simulink model "APP_MyApplication"  (R2018b)
settings: Solver=VariableStepDiscrete  StartTime=0.0  StopTime=10  RelTol=1e-3
PreLoadFcn:
  | if(exist('MBDS_ModelCallback', 'file')), MBDS_ModelCallback('PreLoad'); end;
PostLoadFcn:
  | if(exist('MBDS_ModelCallback', 'file')), MBDS_ModelCallback('PostLoad'); end;
InitFcn:
  | if(exist('MBDS_ModelCallback', 'file')), MBDS_ModelCallback('Init'); end;
StartFcn:
  | if(exist('MBDS_ModelCallback', 'file')), MBDS_ModelCallback('Start'); end;
StopFcn:
  | if(exist('MBDS_ModelCallback', 'file')), MBDS_ModelCallback('Stop'); end;
undefined symbols (not defined in the file): sigbuilder_block, Ts
libraries: KIBES_Signal x499, simulink x8
(part 8 of 10)

== system APP_MyApplication/Model/APP_MyApplication_/EEProm/TimerPulse ==
  note: Timer Pulse
  bo_Enable : Inport  OutDataTypeStr=boolean
  EdgeRising : Subsystem  InitFcn=|  mask(EdgeRising){MBDS_LibraryBlock=on, R_Enabled=off, IV_Enabled=off, IV=0, MBDS_BlockVersion=05.32}
      | if(exist('MBDS_BlockCallback', 'file'))
      |    MBDS_BlockCallback('Update', gcb);
      | end
      mask prompts: MBDS_LibraryBlock "MBDS library block"; R_Enabled "Show R port"; IV_Enabled "Show IV port"; IV "Initial value (IV):"; MBDS_BlockVersion "Block version:"
      mask help: The output indicates true if the input value changes from false to true.
      mask init: same as APP_MyApplication/Model/APP_MyApplication_/OR
      mask Help: eval(['open([workdir(''library_dir:''),''\Blockset\help\'',get_param(gcb,''MaskType''),''.html''])'])
      mask Callback R_Enabled:
      | % Update mask parameter dialog
      | if(exist('MBDS_BlockCallback', 'file'))
      |    MBDS_BlockCallback('R_Enabled', gcb);
      | end
      mask Callback IV_Enabled:
      | % Update mask parameter dialog
      | if(exist('MBDS_BlockCallback', 'file'))
      |    MBDS_BlockCallback('IV_Enabled', gcb);
      | end
      mask Callback IV:
      | % Adopt Value
      | if(exist('MBDS_BlockCallback', 'file'))
      |    MBDS_BlockCallback('IV', gcb);
      | end
      mask DialogControl ParameterTabVar0 Prompt: Main
      mask DialogControl ParameterTabVar01 Prompt: Version
      mask Display:
      | % Show icon or block text
      | if(exist('EdgeRising.tif', 'file'))
      |    image('EdgeRising.tif', [0.295739348370927 0.17 0.378947368421053 0.66]);
      |    disp('')
      | else
      |    disp(sprintf('Rising\nEdge\nDetection'));
      | end
      | 
      | % Display port labels
      | port_label('input', 1, 'u');
      | port_label('output', 1, 'y');
  TimeSource : Subsystem  InitFcn=|  mask(TimeSource){MBDS_LibraryBlock=on, InputValue=10ms, MBDS_BlockVersion=07.21.04}
      | if(exist('MBDS_BlockCallback', 'file'))
      |    MBDS_BlockCallback('Update', gcb);
      | end
      mask prompts: MBDS_LibraryBlock "MBDS Library Block"; InputValue "Constant value:"; MBDS_BlockVersion "Block version:"
      mask help: This block outputs a constant time signal based on a uint32 data type. Specify the time by the 'Constant value' parameter. Comply to the format: 1d2h3m4s5ms, for example 12d10h34m4s231ms, 1s500ms or 2h1s.
      mask init: same as APP_MyApplication/Model/APP_MyApplication_/TimerPulse/TimeSource
      mask Help: eval(['open([workdir(''Library_Dir:''),''\Blockset\Help\'',get_param(gcb,''MaskType''),''.html''])'])
      mask DialogControl ParameterTabVar0 Prompt: Main
      mask DialogControl ParameterTabVar01 Prompt: Version
      mask Display: disp([' ',Text,' ']);
  Timer_RE1 : Subsystem  InitFcn=|  mask(Timer_RE){MBDS_LibraryBlock=on, dT_Enabled=off, dT=1000*Ts, E_Enabled=off, R_Enabled=on, IV_Enabled=on, IV=0, y_Enabled=on, x_Enabled=off, OutDataTypeStr=Inherit: Inherit via back propagation, MBDS_BlockVersion=05.20}
      | if(exist('MBDS_BlockCallback', 'file'))
      |    MBDS_BlockCallback('Update', gcb);
      | end
      mask prompts: MBDS_LibraryBlock "MBDS library block"; dT_Enabled "Show dT port"; dT "Sample rate (dT):"; E_Enabled "Show E port"; R_Enabled "Show R port"; IV_Enabled "Show IV port"; IV "Initial value (IV):"; y_Enabled "Show y port"; x_Enabled "Show x port"; OutDataTypeStr "Output data type:"; MBDS_BlockVersion "Block version:"
      mask help: The block indicates true, if the initial time IV has not passed since the last reset of the block. Reset can only be performed, if the counter has run down to zero.
      mask init: same as APP_MyApplication/Model/APP_MyApplication_/OR
      settings: AttributesFormatString=dT = %<dT>
      mask Help: eval(['open([workdir(''library_dir:''),''\Blockset\help\'',get_param(gcb,''MaskType''),''.html''])'])
      mask Callback dT_Enabled:
      | % Update mask parameter dialog
      | if(exist('MBDS_BlockCallback', 'file'))
      |    MBDS_BlockCallback('dT_Enabled', gcb);
      | end
      mask Callback dT:
      | % Adopt Value
      | if(exist('MBDS_BlockCallback', 'file'))
      |    MBDS_BlockCallback('dT', gcb);
      | end
      mask Callback R_Enabled:
      | % Update mask parameter dialog
      | if(exist('MBDS_BlockCallback', 'file'))
      |    MBDS_BlockCallback('R_Enabled', gcb);
      | end
      mask Callback IV_Enabled:
      | % Update mask parameter dialog
      | if(exist('MBDS_BlockCallback', 'file'))
      |    MBDS_BlockCallback('IV_Enabled', gcb);
      | end
      mask Callback IV:
      | % Adopt Value
      | if(exist('MBDS_BlockCallback', 'file'))
      |    MBDS_BlockCallback('IV', gcb);
      | end
      mask Callback y_Enabled:
      | % Update mask parameter dialog
      | if(exist('MBDS_BlockCallback', 'file'))
      |    MBDS_BlockCallback('y_Enabled', gcb);
      | end
      mask Callback x_Enabled:
      | % Update mask parameter dialog
      | if(exist('MBDS_BlockCallback', 'file'))
      |    MBDS_BlockCallback('x_Enabled', gcb);
      | end
      mask TypeOptions OutDataTypeStr: Inherit: Inherit via back propagation | int8 | uint8 | int16 | uint16 | int32 | uint32
      mask Callback OutDataTypeStr:
      | % Configure data type
      | if(exist('MBDS_BlockCallback', 'file'))
      |    MBDS_BlockCallback('OutDataTypeStr', gcb);
      | end
      mask DialogControl ParameterTabVar0 Prompt: Main
      mask DialogControl ParameterTabVar01 Prompt: Signal Attributes
      mask DialogControl ParameterTabVar012 Prompt: Version
      mask Display:
      | % Show icon or block text
      | if(exist('Timer.tif', 'file'))
      |    image('Timer.tif', [0.295739348370927 0.17 0.378947368421053 0.66]);
      |    disp('')
      | else
      |    disp(sprintf('Timer'));
      | end
      | 
      | % Display port labels
      | port_label('input', 1, 'R');
      | port_label('input', 2, 'IV');
      | port_label('output', 1, 'y');
  bo_Pulse : Outport
  wires:
  EdgeRising/1(y) -> Timer_RE1/1(R)
  Timer_RE1/1(y) -> bo_Pulse/1
  bo_Enable/1 -> EdgeRising/1(u)
  TimeSource/1(Out) -> Timer_RE1/2(IV)

== system APP_MyApplication/Model/APP_MyApplication_/EEProm/TimerPulse1 ==
  note: Timer Pulse
  bo_Enable : Inport  OutDataTypeStr=boolean
  EdgeRising : Subsystem  InitFcn=|  mask(EdgeRising){MBDS_LibraryBlock=on, R_Enabled=off, IV_Enabled=off, IV=0, MBDS_BlockVersion=05.32}
      | if(exist('MBDS_BlockCallback', 'file'))
      |    MBDS_BlockCallback('Update', gcb);
      | end
      mask prompts: MBDS_LibraryBlock "MBDS library block"; R_Enabled "Show R port"; IV_Enabled "Show IV port"; IV "Initial value (IV):"; MBDS_BlockVersion "Block version:"
      mask help: The output indicates true if the input value changes from false to true.
      mask init: same as APP_MyApplication/Model/APP_MyApplication_/OR
      mask Help: eval(['open([workdir(''library_dir:''),''\Blockset\help\'',get_param(gcb,''MaskType''),''.html''])'])
      mask Callback R_Enabled:
      | % Update mask parameter dialog
      | if(exist('MBDS_BlockCallback', 'file'))
      |    MBDS_BlockCallback('R_Enabled', gcb);
      | end
      mask Callback IV_Enabled:
      | % Update mask parameter dialog
      | if(exist('MBDS_BlockCallback', 'file'))
      |    MBDS_BlockCallback('IV_Enabled', gcb);
      | end
      mask Callback IV:
      | % Adopt Value
      | if(exist('MBDS_BlockCallback', 'file'))
      |    MBDS_BlockCallback('IV', gcb);
      | end
      mask DialogControl ParameterTabVar0 Prompt: Main
      mask DialogControl ParameterTabVar01 Prompt: Version
      mask Display:
      | % Show icon or block text
      | if(exist('EdgeRising.tif', 'file'))
      |    image('EdgeRising.tif', [0.295739348370927 0.17 0.378947368421053 0.66]);
      |    disp('')
      | else
      |    disp(sprintf('Rising\nEdge\nDetection'));
      | end
      | 
      | % Display port labels
      | port_label('input', 1, 'u');
      | port_label('output', 1, 'y');
  TimeSource : Subsystem  InitFcn=|  mask(TimeSource){MBDS_LibraryBlock=on, InputValue=10ms, MBDS_BlockVersion=07.21.04}
      | if(exist('MBDS_BlockCallback', 'file'))
      |    MBDS_BlockCallback('Update', gcb);
      | end
      mask prompts: MBDS_LibraryBlock "MBDS Library Block"; InputValue "Constant value:"; MBDS_BlockVersion "Block version:"
      mask help: This block outputs a constant time signal based on a uint32 data type. Specify the time by the 'Constant value' parameter. Comply to the format: 1d2h3m4s5ms, for example 12d10h34m4s231ms, 1s500ms or 2h1s.
      mask init: same as APP_MyApplication/Model/APP_MyApplication_/TimerPulse/TimeSource
      mask Help: eval(['open([workdir(''Library_Dir:''),''\Blockset\Help\'',get_param(gcb,''MaskType''),''.html''])'])
      mask DialogControl ParameterTabVar0 Prompt: Main
      mask DialogControl ParameterTabVar01 Prompt: Version
      mask Display: disp([' ',Text,' ']);
  Timer_RE1 : Subsystem  InitFcn=|  mask(Timer_RE){MBDS_LibraryBlock=on, dT_Enabled=off, dT=1000*Ts, E_Enabled=off, R_Enabled=on, IV_Enabled=on, IV=0, y_Enabled=on, x_Enabled=off, OutDataTypeStr=Inherit: Inherit via back propagation, MBDS_BlockVersion=05.20}
      | if(exist('MBDS_BlockCallback', 'file'))
      |    MBDS_BlockCallback('Update', gcb);
      | end
      mask prompts: MBDS_LibraryBlock "MBDS library block"; dT_Enabled "Show dT port"; dT "Sample rate (dT):"; E_Enabled "Show E port"; R_Enabled "Show R port"; IV_Enabled "Show IV port"; IV "Initial value (IV):"; y_Enabled "Show y port"; x_Enabled "Show x port"; OutDataTypeStr "Output data type:"; MBDS_BlockVersion "Block version:"
      mask help: The block indicates true, if the initial time IV has not passed since the last reset of the block. Reset can only be performed, if the counter has run down to zero.
      mask init: same as APP_MyApplication/Model/APP_MyApplication_/OR
      settings: AttributesFormatString=dT = %<dT>
      mask Help: eval(['open([workdir(''library_dir:''),''\Blockset\help\'',get_param(gcb,''MaskType''),''.html''])'])
      mask Callback dT_Enabled:
      | % Update mask parameter dialog
      | if(exist('MBDS_BlockCallback', 'file'))
      |    MBDS_BlockCallback('dT_Enabled', gcb);
      | end
      mask Callback dT:
      | % Adopt Value
      | if(exist('MBDS_BlockCallback', 'file'))
      |    MBDS_BlockCallback('dT', gcb);
      | end
      mask Callback R_Enabled:
      | % Update mask parameter dialog
      | if(exist('MBDS_BlockCallback', 'file'))
      |    MBDS_BlockCallback('R_Enabled', gcb);
      | end
      mask Callback IV_Enabled:
      | % Update mask parameter dialog
      | if(exist('MBDS_BlockCallback', 'file'))
      |    MBDS_BlockCallback('IV_Enabled', gcb);
      | end
      mask Callback IV:
      | % Adopt Value
      | if(exist('MBDS_BlockCallback', 'file'))
      |    MBDS_BlockCallback('IV', gcb);
      | end
      mask Callback y_Enabled:
      | % Update mask parameter dialog
      | if(exist('MBDS_BlockCallback', 'file'))
      |    MBDS_BlockCallback('y_Enabled', gcb);
      | end
      mask Callback x_Enabled:
      | % Update mask parameter dialog
      | if(exist('MBDS_BlockCallback', 'file'))
      |    MBDS_BlockCallback('x_Enabled', gcb);
      | end
      mask TypeOptions OutDataTypeStr: Inherit: Inherit via back propagation | int8 | uint8 | int16 | uint16 | int32 | uint32
      mask Callback OutDataTypeStr:
      | % Configure data type
      | if(exist('MBDS_BlockCallback', 'file'))
      |    MBDS_BlockCallback('OutDataTypeStr', gcb);
      | end
      mask DialogControl ParameterTabVar0 Prompt: Main
      mask DialogControl ParameterTabVar01 Prompt: Signal Attributes
      mask DialogControl ParameterTabVar012 Prompt: Version
      mask Display:
      | % Show icon or block text
      | if(exist('Timer.tif', 'file'))
      |    image('Timer.tif', [0.295739348370927 0.17 0.378947368421053 0.66]);
      |    disp('')
      | else
      |    disp(sprintf('Timer'));
      | end
      | 
      | % Display port labels
      | port_label('input', 1, 'R');
      | port_label('input', 2, 'IV');
      | port_label('output', 1, 'y');
  bo_Pulse : Outport
  wires:
  EdgeRising/1(y) -> Timer_RE1/1(R)
  Timer_RE1/1(y) -> bo_Pulse/1
  bo_Enable/1 -> EdgeRising/1(u)
  TimeSource/1(Out) -> Timer_RE1/2(IV)

== system APP_MyApplication/Model/APP_MyApplication_/TimerPulse/EdgeRising ==
  note: EdgeRising
  u : Inport  OutDataTypeStr=boolean
  Data Type Duplicate : DataTypeDuplicate
  IV : Constant  Value=0  OutDataTypeStr=Inherit: Inherit via back propagation
  NoReset : Subsystem
  R : Constant  Value=0  OutDataTypeStr=boolean
  Relational Operator : RelationalOperator  Operator=<  OutDataTypeStr=boolean  RndMeth=Nearest  InputSameDT=on
  Unit Delay : UnitDelay  SampleTime=-1
  y : Outport
  wires:
  IV/1 -> NoReset/1(Unused1), Data Type Duplicate/2
  u/1 -> Unit Delay/1, Relational Operator/2, Data Type Duplicate/1
  R/1 -> NoReset/2(Unused2)
  NoReset/1(y) -> Relational Operator/1
  Unit Delay/1 -> NoReset/3(u)
  Relational Operator/1 -> y/1

== system APP_MyApplication/Model/APP_MyApplication_/TimerPulse/TimeSource ==
  note: TimeSource
  Constant : Constant  Value=Value  OutDataTypeStr=uint32  LockScale=on
  Out : Outport
  wires:
  Constant/1 -> Out/1

== system APP_MyApplication/Model/APP_MyApplication_/TimerPulse/Timer_RE1 ==
  note: Timer_RE
  R : Inport  OutDataTypeStr=boolean
  IV : Inport  Port=2
  Constant : Constant  Value=0  OutDataTypeStr=Inherit: Inherit via back propagation
  Constant1 : Constant  Value=0  OutDataTypeStr=Inherit: Inherit via back propagation
  Constant2 : Constant  Value=0  OutDataTypeStr=Inherit: Inherit via back propagation
  Data Type Duplicate : DataTypeDuplicate  NumInputPorts=3
  DoubleReset : Subsystem
  E : Constant  OutDataTypeStr=boolean
  NoEnable : Subsystem
  Relational Operator : RelationalOperator  Operator=<=  OutDataTypeStr=boolean  RndMeth=Nearest
  Relational Operator1 : RelationalOperator  Operator=>  OutDataTypeStr=boolean  RndMeth=Nearest
  Relational Operator2 : RelationalOperator  Operator=>  OutDataTypeStr=boolean  RndMeth=Nearest  InputSameDT=on
  Subtract : Sum  Inputs=+-  OutDataTypeStr=Inherit: Inherit via back propagation
  Switch1 : Switch  Criteria=u2 ~= 0  OutDataTypeStr=Inherit: Inherit via back propagation
  Unit Delay : UnitDelay  SampleTime=-1
  dT : Constant  Value=1000*Ts  OutDataTypeStr=Inherit: Inherit via back propagation
  x : Terminator
  y : Outport
  wires:
  R/1 -> DoubleReset/2(R1)
  E/1 -> NoEnable/2(Unused1)
  IV/1 -> Data Type Duplicate/1, DoubleReset/1(IV)
  Relational Operator/1 -> DoubleReset/3(R2)
  DoubleReset/1(y) -> Relational Operator2/1, Unit Delay/1, x/1, Data Type Duplicate/3
  Constant2/1 -> Relational Operator2/2
  Constant/1 -> Switch1/3
  Subtract/1 -> Switch1/1
  Relational Operator1/1 -> Switch1/2
  Switch1/1 -> NoEnable/1(u)
  dT/1 -> Subtract/2, Relational Operator1/2
  Unit Delay/1 -> NoEnable/3(Unused2), Relational Operator1/1, Subtract/1, Relational Operator/1, Data Type Duplicate/2
  Constant1/1 -> Relational Operator/2
  NoEnable/1(y) -> DoubleReset/4(u)
  Relational Operator2/1 -> y/1

== system APP_MyApplication/Model/APP_MyApplication_/UDS Service/RSFlipFlop ==
  note: RSFlipFlop
  SET : Inport  OutDataTypeStr=boolean
  RST : Inport  Port=2  OutDataTypeStr=boolean
  Constant : Constant  Value=0  OutDataTypeStr=Inherit: Inherit via back propagation
  Constant1 : Constant  OutDataTypeStr=Inherit: Inherit via back propagation
  Data Type Duplicate : DataTypeDuplicate  NumInputPorts=3
  Logical Operator : Logic  Operator=NOT  AllPortsSameDT=off  OutDataTypeStr=boolean
  Switch1 : Switch  Criteria=u2 ~= 0  OutDataTypeStr=Inherit: Inherit via back propagation
  Switch2 : Switch  Criteria=u2 ~= 0  OutDataTypeStr=Inherit: Inherit via back propagation
  Unit Delay : UnitDelay  SampleTime=-1
  Q : Outport
  ~Q : Outport  Port=2
  wires:
  Switch1/1 -> Q/1, Data Type Duplicate/3, Unit Delay/1, Logical Operator/1
  Constant/1 -> Switch1/1
  RST/1 -> Data Type Duplicate/2, Switch1/2
  SET/1 -> Data Type Duplicate/1, Switch2/2
  Constant1/1 -> Switch2/1
  Switch2/1 -> Switch1/3
  Logical Operator/1 -> ~Q/1
  Unit Delay/1 -> Switch2/3

== system APP_MyApplication/Model/APP_MyApplication_/DTC/DateTimeDisassemble/CheckIfTimeDataIsValid ==
  note: 2099-12-31-23:59:59
  note: Check if time data is valid
  u32_DateTime : Inport  OutDataTypeStr=uint32
  Constant14 : Constant  Value=4102444799  OutDataTypeStr=uint32
  Relational Operator : RelationalOperator  Operator=<=  OutDataTypeStr=boolean  RndMeth=Nearest
  bo_ENO : Outport  OutDataTypeStr=boolean
  wires:
  Constant14/1 -> Relational Operator/2
  u32_DateTime/1 -> Relational Operator/1
  Relational Operator/1 -> bo_ENO/1

== system APP_MyApplication/Model/APP_MyApplication_/DTC/DateTimeDisassemble/CheckLeapYearsAndRemainingDays ==
  note: Year
  note: Check leap year and calculate remaining days in current year
  note: avoid overflow
  u16_NrOfDays : Inport  OutDataTypeStr=uint16
  Add3 : Sum  Inputs=++-  OutDataTypeStr=uint16
  CalculateLeapYearsSince1970 : Subsystem
  CalculateRemainingDays : Subsystem
  CheckIfCorrectedTempYearIsLeap : Subsystem
  CheckIfTempYearIsCorrect : Subsystem
  CheckLeapYear : Subsystem
  Constant2 : Constant  OutDataTypeStr=uint16
  Constant6 : Constant  Value=0  OutDataTypeStr=uint16
  DaysPerNonLeapYear : Constant  Value=365  OutDataTypeStr=uint16
  Math Function3 : Math  Operator=rem  OutputSignalType=real  SaturateOnIntegerOverflow=on
  Relational Operator1 : RelationalOperator  Operator===  OutDataTypeStr=boolean  RndMeth=Nearest  InputSameDT=on
  Switch1 : Switch  Criteria=u2 ~= 0  OutDataTypeStr=uint16
  u16_TempDate : Outport  OutDataTypeStr=uint16
  u16_Year : Outport  Port=2  OutDataTypeStr=uint16
  bo_LeapYear : Outport  Port=3  OutDataTypeStr=boolean
  wires:
  u16_NrOfDays/1 -> CalculateLeapYearsSince1970/1(u16_NrOfDays), Math Function3/1
  DaysPerNonLeapYear/1 -> CalculateRemainingDays/5(u16_DaysPerCommonYear), Math Function3/2, CalculateLeapYearsSince1970/2(u16_DaysPerCommonYear)
  Math Function3/1 -> CalculateRemainingDays/3(u16_TempRemainingDays), CheckIfTempYearIsCorrect/1(u16_TempRemainingDays)
  Switch1/1 -> CheckLeapYear/1(u16_Year), u16_Year/1
  CalculateLeapYearsSince1970/2(u16_TempYear) -> Switch1/1, Add3/2, Relational Operator1/2
  Add3/1 -> Switch1/3, CheckIfCorrectedTempYearIsLeap/1(u16_CorrectedTempYear)
  CheckLeapYear/1(bo_LeapYear) -> bo_LeapYear/1
  Constant6/1 -> Relational Operator1/1
  Constant2/1 -> Add3/3
  Relational Operator1/1 -> Add3/1
  CalculateLeapYearsSince1970/1(u16_NrOfLeapYears) -> [u16_NrOfLeapYears]
  [u16_NrOfLeapYears] -> CheckIfTempYearIsCorrect/2(u16_NrOfLeapYears)
  CheckIfTempYearIsCorrect/1(bo_IsTempYearCorrect) -> Switch1/2, CalculateRemainingDays/2(bo_IsTempYearCorrect)
  CalculateRemainingDays/1(u16_TempDate) -> u16_TempDate/1
  CheckIfCorrectedTempYearIsLeap/1(bo_IsCorrectedYearLeapYear) -> CalculateRemainingDays/1(bo_IsCorrectedYearLeapYear)
  [u16_NrOfLeapYears] -> CalculateRemainingDays/4(u16_NrOfLeapYears)

== system APP_MyApplication/Model/APP_MyApplication_/DTC/DateTimeDisassemble/ConvertToDayOfWeek ==
  note: 1970-01-01 is Thursday
  note: Convert to day of week
  u16_NrOfDays : Inport  OutDataTypeStr=uint16
  Add2 : Sum  OutDataTypeStr=uint16
  Add3 : Sum  OutDataTypeStr=uint16
  Constant3 : Constant  Value=7  OutDataTypeStr=uint16
  Constant4 : Constant  Value=3  OutDataTypeStr=uint8
  Constant5 : Constant  OutDataTypeStr=uint8
  Data Type Conversion3 : DataTypeConversion  OutDataTypeStr=uint8
  Math Function : Math  Operator=rem  OutputSignalType=real  SaturateOnIntegerOverflow=on
  u8_DayOfWeek : Outport  OutDataTypeStr=uint8
  wires:
  Data Type Conversion3/1 -> u8_DayOfWeek/1
  Constant5/1 -> Add3/2
  Constant3/1 -> Math Function/2
  Constant4/1 -> Add2/2
  Add2/1 -> Math Function/1
  Math Function/1 -> Add3/1
  Add3/1 -> Data Type Conversion3/1
  u16_NrOfDays/1 -> Add2/1

== system APP_MyApplication/Model/APP_MyApplication_/DTC/DateTimeDisassemble/ConvertToMonthAndDay ==
  note: Days per month
  note: Count number of cycles (= Month - 1)
  note: Check if there are less days remaining than the next month has
  note: Convert to month and day
  u16_TempDate : Inport  OutDataTypeStr=uint16
  bo_LeapYear : Inport  Port=2  OutDataTypeStr=boolean
  Add5 : Sum  OutDataTypeStr=uint8
  CheckNrOfDaysInNextMonth : Subsystem
  Constant1 : Constant  Value=[0 31 28 31 30 31 30 31 31 30 31 30 31]  OutDataTypeStr=uint8
  Data Type Conversion : DataTypeConversion  OutDataTypeStr=uint8
  Data Type Conversion1 : DataTypeConversion  OutDataTypeStr=uint16
  Relational Operator1 : RelationalOperator  OutDataTypeStr=boolean  RndMeth=Nearest  InputSameDT=on
  SubstractDaysOfMonths : Subsystem
  Unit Delay1 : UnitDelay  SampleTime=-1
  While Iterator : WhileIterator  MaxIters=12  WhileBlockType=do-while  ResetStates=reset  ShowIterationPort=on  OutputDataType=int8
  u8_MonthMinusOne : Outport  OutDataTypeStr=uint8
  u16_DayMinusOne : Outport  Port=2  OutDataTypeStr=uint16
  wires:
  bo_LeapYear/1 -> SubstractDaysOfMonths/2(bo_LeapYear), CheckNrOfDaysInNextMonth/3(bo_LeapYear)
  Relational Operator1/1 -> Data Type Conversion/1, While Iterator/1
  While Iterator/1 -> SubstractDaysOfMonths/3(i8_IterationNr), CheckNrOfDaysInNextMonth/2(i8_IterationNr)
  Add5/1 -> u8_MonthMinusOne/1, Unit Delay1/1
  Unit Delay1/1 -> Add5/2
  Data Type Conversion/1 -> Add5/1
  SubstractDaysOfMonths/1(u16_RemainingDays) -> u16_DayMinusOne/1, Relational Operator1/1
  CheckNrOfDaysInNextMonth/1(u8_DaysInNextMonth) -> Data Type Conversion1/1
  u16_TempDate/1 -> SubstractDaysOfMonths/1(u16_TempDate)
  Constant1/1 -> SubstractDaysOfMonths/4(u8_DaysPerMonth), CheckNrOfDaysInNextMonth/1(u8_DaysPerMonth)
  Data Type Conversion1/1 -> Relational Operator1/2

== system APP_MyApplication/Model/APP_MyApplication_/DTC/DateTimeDisassemble/ConvertToTimeAndNrOfDays ==
  note: Convert date time to time and number of days
  u32_DateTime : Inport  OutDataTypeStr=uint32
  CalculateHours : Subsystem
  CalculateMinutes : Subsystem
  CalculateSeconds : Subsystem
  u8_Seconds : Outport  OutDataTypeStr=uint8
  u8_Minutes : Outport  Port=2  OutDataTypeStr=uint8
  u8_Hours : Outport  Port=3  OutDataTypeStr=uint8
  u16_NrOfDays : Outport  Port=4  OutDataTypeStr=uint16
  wires:
  CalculateSeconds/1(u8_Seconds) -> u8_Seconds/1
  CalculateHours/2(u16_NrOfDays) -> u16_NrOfDays/1
  u32_DateTime/1 -> CalculateSeconds/1(u32_TimeInSeconds)
  CalculateSeconds/2(u32_TempDateMin) -> CalculateMinutes/1(u32_TempDateMin)
  CalculateMinutes/1(u8_Minutes) -> u8_Minutes/1
  CalculateMinutes/2(u32_TempDateHrs) -> CalculateHours/1(u32_TempDateHrs)
  CalculateHours/1(u8_Hours) -> u8_Hours/1

== system APP_MyApplication/Model/APP_MyApplication_/DTC/GetBit/LoopOverBits ==
  note: Generate bit mask
  note: Determine bit value
  note: No saturation
      | needed !
  u : Inport
  SEL : Inport  Port=2
  Assignment1 : Assignment  IndexMode=Zero-based  IndexOptions=Index vector (port)  Indices=1  OutputSizes=[1 1]
  Bitwise Operator1 : simulink/Logic and Bit Operations/Bitwise Operator  logicop=AND  UseBitMask=off  NumInputPorts=2  BitMask=bin2dec('11011001')  BitMaskRealWorld=Stored Integer
  Constant2 : Constant  Value=0  OutDataTypeStr=Inherit: Inherit via back propagation
  Constant3 : Constant  OutDataTypeStr=Inherit: Inherit via back propagation
  Data Type Duplicate : DataTypeDuplicate  InitFcn=|
      | try
      |    MBDS_BlockCallback('Update', gcb);
      | end
  DataType : DataTypeConversion  OutDataTypeStr=boolean
  DataType1 : DataTypeConversion  OutDataTypeStr=uint8
  For Iterator : ForIterator  IterationSource=external  IndexMode=Zero-based  IterationVariableDataType=int8
  IndexOffset : Constant  Value=0  OutDataTypeStr=Inherit: Inherit via back propagation
  Relational Operator : RelationalOperator  Operator=~=  OutDataTypeStr=boolean  RndMeth=Nearest
  Selector : Selector  IndexMode=Zero-based  IndexOptions=Index vector (port)  Indices=[1 3]  OutputSizes=1
  Shift Arithmetic : ArithShift  BitShiftNumberSource=Input port  BitShiftNumber=8  BitShiftDirection=Left
      settings: InputPortMap=u0,p1
  Subtract : Sum  Inputs=+-  OutDataTypeStr=Inherit: Inherit via back propagation  InputSameDT=on
  Width : Width  DataType=uint8
  y : Outport
  wires:
  IndexOffset/1 -> Subtract/2
  Subtract/1 -> Shift Arithmetic/2
  Selector/1 -> Subtract/1
  For Iterator/1 -> Selector/2, Assignment1/3
  Width/1 -> For Iterator/1
  Constant3/1 -> Shift Arithmetic/1, Data Type Duplicate/2
  Shift Arithmetic/1 -> Bitwise Operator1/2
  Bitwise Operator1/1 -> Relational Operator/1
  Constant2/1 -> Relational Operator/2
  Relational Operator/1 -> Assignment1/2
  Assignment1/1 -> y/1
  DataType/1 -> Assignment1/1
  SEL/1 -> DataType1/1, DataType/1, Width/1
  DataType1/1 -> Selector/1
  u/1 -> Bitwise Operator1/1, Data Type Duplicate/1

== system APP_MyApplication/Model/APP_MyApplication_/DTC/GetBit1/LoopOverBits ==
  note: Generate bit mask
  note: Determine bit value
  note: No saturation
      | needed !
  u : Inport
  SEL : Inport  Port=2
  Assignment1 : Assignment  IndexMode=Zero-based  IndexOptions=Index vector (port)  Indices=1  OutputSizes=[1 1]
  Bitwise Operator1 : simulink/Logic and Bit Operations/Bitwise Operator  logicop=AND  UseBitMask=off  NumInputPorts=2  BitMask=bin2dec('11011001')  BitMaskRealWorld=Stored Integer
  Constant2 : Constant  Value=0  OutDataTypeStr=Inherit: Inherit via back propagation
  Constant3 : Constant  OutDataTypeStr=Inherit: Inherit via back propagation
  Data Type Duplicate : DataTypeDuplicate  InitFcn=|
      | try
      |    MBDS_BlockCallback('Update', gcb);
      | end
  DataType : DataTypeConversion  OutDataTypeStr=boolean
  DataType1 : DataTypeConversion  OutDataTypeStr=uint8
  For Iterator : ForIterator  IterationSource=external  IndexMode=Zero-based  IterationVariableDataType=int8
  IndexOffset : Constant  Value=0  OutDataTypeStr=Inherit: Inherit via back propagation
  Relational Operator : RelationalOperator  Operator=~=  OutDataTypeStr=boolean  RndMeth=Nearest
  Selector : Selector  IndexMode=Zero-based  IndexOptions=Index vector (port)  Indices=[1 3]  OutputSizes=1
  Shift Arithmetic : ArithShift  BitShiftNumberSource=Input port  BitShiftNumber=8  BitShiftDirection=Left
      settings: InputPortMap=u0,p1
  Subtract : Sum  Inputs=+-  OutDataTypeStr=Inherit: Inherit via back propagation  InputSameDT=on
  Width : Width  DataType=uint8
  y : Outport
  wires:
  IndexOffset/1 -> Subtract/2
  Subtract/1 -> Shift Arithmetic/2
  Selector/1 -> Subtract/1
  For Iterator/1 -> Selector/2, Assignment1/3
  Width/1 -> For Iterator/1
  Constant3/1 -> Shift Arithmetic/1, Data Type Duplicate/2
  Shift Arithmetic/1 -> Bitwise Operator1/2
  Bitwise Operator1/1 -> Relational Operator/1
  Constant2/1 -> Relational Operator/2
  Relational Operator/1 -> Assignment1/2
  Assignment1/1 -> y/1
  DataType/1 -> Assignment1/1
  SEL/1 -> DataType1/1, DataType/1, Width/1
  DataType1/1 -> Selector/1
  u/1 -> Bitwise Operator1/1, Data Type Duplicate/1

== system APP_MyApplication/Model/APP_MyApplication_/DTC/GetBit2/LoopOverBits ==
  note: Generate bit mask
  note: Determine bit value
  note: No saturation
      | needed !
  u : Inport
  SEL : Inport  Port=2
  Assignment1 : Assignment  IndexMode=Zero-based  IndexOptions=Index vector (port)  Indices=1  OutputSizes=[1 1]
  Bitwise Operator1 : simulink/Logic and Bit Operations/Bitwise Operator  logicop=AND  UseBitMask=off  NumInputPorts=2  BitMask=bin2dec('11011001')  BitMaskRealWorld=Stored Integer
  Constant2 : Constant  Value=0  OutDataTypeStr=Inherit: Inherit via back propagation
  Constant3 : Constant  OutDataTypeStr=Inherit: Inherit via back propagation
  Data Type Duplicate : DataTypeDuplicate  InitFcn=|
      | try
      |    MBDS_BlockCallback('Update', gcb);
      | end
  DataType : DataTypeConversion  OutDataTypeStr=boolean
  DataType1 : DataTypeConversion  OutDataTypeStr=uint8
  For Iterator : ForIterator  IterationSource=external  IndexMode=Zero-based  IterationVariableDataType=int8
  IndexOffset : Constant  Value=0  OutDataTypeStr=Inherit: Inherit via back propagation
  Relational Operator : RelationalOperator  Operator=~=  OutDataTypeStr=boolean  RndMeth=Nearest
  Selector : Selector  IndexMode=Zero-based  IndexOptions=Index vector (port)  Indices=[1 3]  OutputSizes=1
  Shift Arithmetic : ArithShift  BitShiftNumberSource=Input port  BitShiftNumber=8  BitShiftDirection=Left
      settings: InputPortMap=u0,p1
  Subtract : Sum  Inputs=+-  OutDataTypeStr=Inherit: Inherit via back propagation  InputSameDT=on
  Width : Width  DataType=uint8
  y : Outport
  wires:
  IndexOffset/1 -> Subtract/2
  Subtract/1 -> Shift Arithmetic/2
  Selector/1 -> Subtract/1
  For Iterator/1 -> Selector/2, Assignment1/3
  Width/1 -> For Iterator/1
  Constant3/1 -> Shift Arithmetic/1, Data Type Duplicate/2
  Shift Arithmetic/1 -> Bitwise Operator1/2
  Bitwise Operator1/1 -> Relational Operator/1
  Constant2/1 -> Relational Operator/2
  Relational Operator/1 -> Assignment1/2
  Assignment1/1 -> y/1
  DataType/1 -> Assignment1/1
  SEL/1 -> DataType1/1, DataType/1, Width/1
  DataType1/1 -> Selector/1
  u/1 -> Bitwise Operator1/1, Data Type Duplicate/1

== system APP_MyApplication/Model/APP_MyApplication_/DTC/GetBit3/LoopOverBits ==
  note: Generate bit mask
  note: Determine bit value
  note: No saturation
      | needed !
  u : Inport
  SEL : Inport  Port=2
  Assignment1 : Assignment  IndexMode=Zero-based  IndexOptions=Index vector (port)  Indices=1  OutputSizes=[1 1]
  Bitwise Operator1 : simulink/Logic and Bit Operations/Bitwise Operator  logicop=AND  UseBitMask=off  NumInputPorts=2  BitMask=bin2dec('11011001')  BitMaskRealWorld=Stored Integer
  Constant2 : Constant  Value=0  OutDataTypeStr=Inherit: Inherit via back propagation
  Constant3 : Constant  OutDataTypeStr=Inherit: Inherit via back propagation
  Data Type Duplicate : DataTypeDuplicate  InitFcn=|
      | try
      |    MBDS_BlockCallback('Update', gcb);
      | end
  DataType : DataTypeConversion  OutDataTypeStr=boolean
  DataType1 : DataTypeConversion  OutDataTypeStr=uint8
  For Iterator : ForIterator  IterationSource=external  IndexMode=Zero-based  IterationVariableDataType=int8
  IndexOffset : Constant  Value=0  OutDataTypeStr=Inherit: Inherit via back propagation
  Relational Operator : RelationalOperator  Operator=~=  OutDataTypeStr=boolean  RndMeth=Nearest
  Selector : Selector  IndexMode=Zero-based  IndexOptions=Index vector (port)  Indices=[1 3]  OutputSizes=1
  Shift Arithmetic : ArithShift  BitShiftNumberSource=Input port  BitShiftNumber=8  BitShiftDirection=Left
      settings: InputPortMap=u0,p1
  Subtract : Sum  Inputs=+-  OutDataTypeStr=Inherit: Inherit via back propagation  InputSameDT=on
  Width : Width  DataType=uint8
  y : Outport
  wires:
  IndexOffset/1 -> Subtract/2
  Subtract/1 -> Shift Arithmetic/2
  Selector/1 -> Subtract/1
  For Iterator/1 -> Selector/2, Assignment1/3
  Width/1 -> For Iterator/1
  Constant3/1 -> Shift Arithmetic/1, Data Type Duplicate/2
  Shift Arithmetic/1 -> Bitwise Operator1/2
  Bitwise Operator1/1 -> Relational Operator/1
  Constant2/1 -> Relational Operator/2
  Relational Operator/1 -> Assignment1/2
  Assignment1/1 -> y/1
  DataType/1 -> Assignment1/1
  SEL/1 -> DataType1/1, DataType/1, Width/1
  DataType1/1 -> Selector/1
  u/1 -> Bitwise Operator1/1, Data Type Duplicate/1

== system APP_MyApplication/Model/APP_MyApplication_/DTC/GetBit4/LoopOverBits ==
  note: Generate bit mask
  note: Determine bit value
  note: No saturation
      | needed !
  u : Inport
  SEL : Inport  Port=2
  Assignment1 : Assignment  IndexMode=Zero-based  IndexOptions=Index vector (port)  Indices=1  OutputSizes=[1 1]
  Bitwise Operator1 : simulink/Logic and Bit Operations/Bitwise Operator  logicop=AND  UseBitMask=off  NumInputPorts=2  BitMask=bin2dec('11011001')  BitMaskRealWorld=Stored Integer
  Constant2 : Constant  Value=0  OutDataTypeStr=Inherit: Inherit via back propagation
  Constant3 : Constant  OutDataTypeStr=Inherit: Inherit via back propagation
  Data Type Duplicate : DataTypeDuplicate  InitFcn=|
      | try
      |    MBDS_BlockCallback('Update', gcb);
      | end
  DataType : DataTypeConversion  OutDataTypeStr=boolean
  DataType1 : DataTypeConversion  OutDataTypeStr=uint8
  For Iterator : ForIterator  IterationSource=external  IndexMode=Zero-based  IterationVariableDataType=int8
  IndexOffset : Constant  Value=0  OutDataTypeStr=Inherit: Inherit via back propagation
  Relational Operator : RelationalOperator  Operator=~=  OutDataTypeStr=boolean  RndMeth=Nearest
  Selector : Selector  IndexMode=Zero-based  IndexOptions=Index vector (port)  Indices=[1 3]  OutputSizes=1
  Shift Arithmetic : ArithShift  BitShiftNumberSource=Input port  BitShiftNumber=8  BitShiftDirection=Left
      settings: InputPortMap=u0,p1
  Subtract : Sum  Inputs=+-  OutDataTypeStr=Inherit: Inherit via back propagation  InputSameDT=on
  Width : Width  DataType=uint8
  y : Outport
  wires:
  IndexOffset/1 -> Subtract/2
  Subtract/1 -> Shift Arithmetic/2
  Selector/1 -> Subtract/1
  For Iterator/1 -> Selector/2, Assignment1/3
  Width/1 -> For Iterator/1
  Constant3/1 -> Shift Arithmetic/1, Data Type Duplicate/2
  Shift Arithmetic/1 -> Bitwise Operator1/2
  Bitwise Operator1/1 -> Relational Operator/1
  Constant2/1 -> Relational Operator/2
  Relational Operator/1 -> Assignment1/2
  Assignment1/1 -> y/1
  DataType/1 -> Assignment1/1
  SEL/1 -> DataType1/1, DataType/1, Width/1
  DataType1/1 -> Selector/1
  u/1 -> Bitwise Operator1/1, Data Type Duplicate/1

== system APP_MyApplication/Model/APP_MyApplication_/DTC/GetBit5/LoopOverBits ==
  note: Generate bit mask
  note: Determine bit value
  note: No saturation
      | needed !
  u : Inport
  SEL : Inport  Port=2
  Assignment1 : Assignment  IndexMode=Zero-based  IndexOptions=Index vector (port)  Indices=1  OutputSizes=[1 1]
  Bitwise Operator1 : simulink/Logic and Bit Operations/Bitwise Operator  logicop=AND  UseBitMask=off  NumInputPorts=2  BitMask=bin2dec('11011001')  BitMaskRealWorld=Stored Integer
  Constant2 : Constant  Value=0  OutDataTypeStr=Inherit: Inherit via back propagation
  Constant3 : Constant  OutDataTypeStr=Inherit: Inherit via back propagation
  Data Type Duplicate : DataTypeDuplicate  InitFcn=|
      | try
      |    MBDS_BlockCallback('Update', gcb);
      | end
  DataType : DataTypeConversion  OutDataTypeStr=boolean
  DataType1 : DataTypeConversion  OutDataTypeStr=uint8
  For Iterator : ForIterator  IterationSource=external  IndexMode=Zero-based  IterationVariableDataType=int8
  IndexOffset : Constant  Value=0  OutDataTypeStr=Inherit: Inherit via back propagation
  Relational Operator : RelationalOperator  Operator=~=  OutDataTypeStr=boolean  RndMeth=Nearest
  Selector : Selector  IndexMode=Zero-based  IndexOptions=Index vector (port)  Indices=[1 3]  OutputSizes=1
  Shift Arithmetic : ArithShift  BitShiftNumberSource=Input port  BitShiftNumber=8  BitShiftDirection=Left
      settings: InputPortMap=u0,p1
  Subtract : Sum  Inputs=+-  OutDataTypeStr=Inherit: Inherit via back propagation  InputSameDT=on
  Width : Width  DataType=uint8
  y : Outport
  wires:
  IndexOffset/1 -> Subtract/2
  Subtract/1 -> Shift Arithmetic/2
  Selector/1 -> Subtract/1
  For Iterator/1 -> Selector/2, Assignment1/3
  Width/1 -> For Iterator/1
  Constant3/1 -> Shift Arithmetic/1, Data Type Duplicate/2
  Shift Arithmetic/1 -> Bitwise Operator1/2
  Bitwise Operator1/1 -> Relational Operator/1
  Constant2/1 -> Relational Operator/2
  Relational Operator/1 -> Assignment1/2
  Assignment1/1 -> y/1
  DataType/1 -> Assignment1/1
  SEL/1 -> DataType1/1, DataType/1, Width/1
  DataType1/1 -> Selector/1
  u/1 -> Bitwise Operator1/1, Data Type Duplicate/1

== system APP_MyApplication/Model/APP_MyApplication_/DTC/GetBit6/LoopOverBits ==
  note: Generate bit mask
  note: Determine bit value
  note: No saturation
      | needed !
  u : Inport
  SEL : Inport  Port=2
  Assignment1 : Assignment  IndexMode=Zero-based  IndexOptions=Index vector (port)  Indices=1  OutputSizes=[1 1]
  Bitwise Operator1 : simulink/Logic and Bit Operations/Bitwise Operator  logicop=AND  UseBitMask=off  NumInputPorts=2  BitMask=bin2dec('11011001')  BitMaskRealWorld=Stored Integer
  Constant2 : Constant  Value=0  OutDataTypeStr=Inherit: Inherit via back propagation
  Constant3 : Constant  OutDataTypeStr=Inherit: Inherit via back propagation
  Data Type Duplicate : DataTypeDuplicate  InitFcn=|
      | try
      |    MBDS_BlockCallback('Update', gcb);
      | end
  DataType : DataTypeConversion  OutDataTypeStr=boolean
  DataType1 : DataTypeConversion  OutDataTypeStr=uint8
  For Iterator : ForIterator  IterationSource=external  IndexMode=Zero-based  IterationVariableDataType=int8
  IndexOffset : Constant  Value=0  OutDataTypeStr=Inherit: Inherit via back propagation
  Relational Operator : RelationalOperator  Operator=~=  OutDataTypeStr=boolean  RndMeth=Nearest
  Selector : Selector  IndexMode=Zero-based  IndexOptions=Index vector (port)  Indices=[1 3]  OutputSizes=1
  Shift Arithmetic : ArithShift  BitShiftNumberSource=Input port  BitShiftNumber=8  BitShiftDirection=Left
      settings: InputPortMap=u0,p1
  Subtract : Sum  Inputs=+-  OutDataTypeStr=Inherit: Inherit via back propagation  InputSameDT=on
  Width : Width  DataType=uint8
  y : Outport
  wires:
  IndexOffset/1 -> Subtract/2
  Subtract/1 -> Shift Arithmetic/2
  Selector/1 -> Subtract/1
  For Iterator/1 -> Selector/2, Assignment1/3
  Width/1 -> For Iterator/1
  Constant3/1 -> Shift Arithmetic/1, Data Type Duplicate/2
  Shift Arithmetic/1 -> Bitwise Operator1/2
  Bitwise Operator1/1 -> Relational Operator/1
  Constant2/1 -> Relational Operator/2
  Relational Operator/1 -> Assignment1/2
  Assignment1/1 -> y/1
  DataType/1 -> Assignment1/1
  SEL/1 -> DataType1/1, DataType/1, Width/1
  DataType1/1 -> Selector/1
  u/1 -> Bitwise Operator1/1, Data Type Duplicate/1

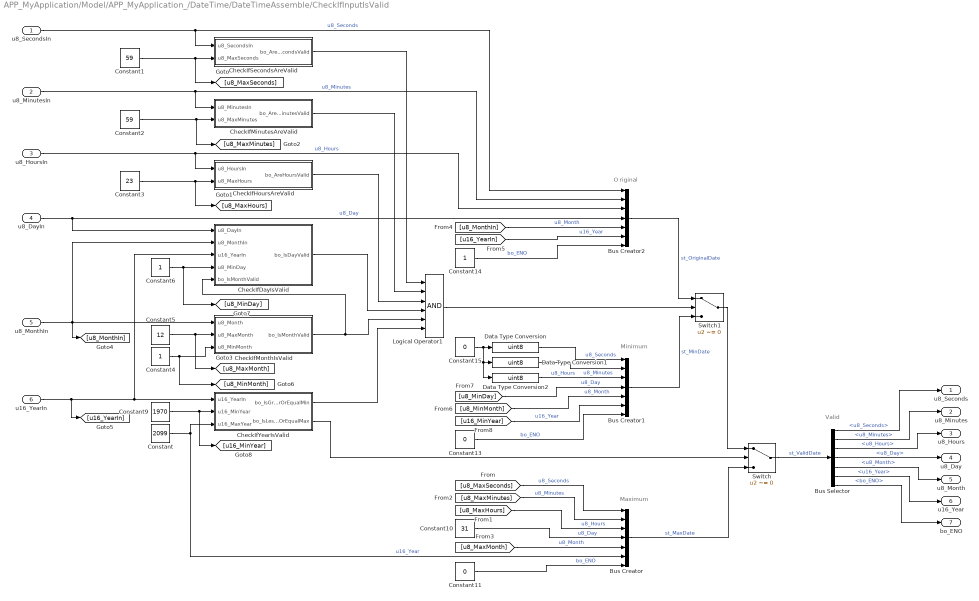
== system APP_MyApplication/Model/APP_MyApplication_/DateTime/DateTimeAssemble/CheckIfInputIsValid ==
  note: Valid
  note: O riginal
  note: Minimum
  note: Maximum
  u8_SecondsIn : Inport  OutDataTypeStr=uint8
  u8_MinutesIn : Inport  Port=2  OutDataTypeStr=uint8
  u8_HoursIn : Inport  Port=3  OutDataTypeStr=uint8
  u8_DayIn : Inport  Port=4  OutDataTypeStr=uint8
  u8_MonthIn : Inport  Port=5  OutDataTypeStr=uint8
  u16_YearIn : Inport  Port=6  OutDataTypeStr=uint16
  Bus Creator : BusCreator  Inputs='u8_Seconds','u8_Minutes','u8_Hours','u8_Day','u8_Month','u16_Year','bo_ENO'
  Bus Creator1 : BusCreator  Inputs='u8_Seconds','u8_Minutes','u8_Hours','u8_Day','u8_Month','u16_Year','bo_ENO'
  Bus Creator2 : BusCreator  Inputs='u8_Seconds','u8_Minutes','u8_Hours','u8_Day','u8_Month','u16_Year','bo_ENO'
  Bus Selector : BusSelector  OutputSignals=u8_Seconds,u8_Minutes,u8_Hours,u8_Day,u8_Month,u16_Year,bo_ENO
  CheckIfDayIsValid : Subsystem
  CheckIfHoursAreValid : Subsystem
  CheckIfMinutesAreValid : Subsystem
  CheckIfMonthIsValid : Subsystem
  CheckIfSecondsAreValid : Subsystem
  CheckIfYearIsValid : Subsystem
  Constant : Constant  Value=2099  OutDataTypeStr=uint16
  Constant1 : Constant  Value=59  OutDataTypeStr=uint8
  Constant10 : Constant  Value=31  OutDataTypeStr=uint8
  Constant11 : Constant  Value=0  OutDataTypeStr=boolean
  Constant13 : Constant  Value=0  OutDataTypeStr=boolean
  Constant14 : Constant  OutDataTypeStr=boolean
  Constant15 : Constant  Value=0  OutDataTypeStr=uint8
  Constant2 : Constant  Value=59  OutDataTypeStr=uint8
  Constant3 : Constant  Value=23  OutDataTypeStr=uint8
  Constant4 : Constant  OutDataTypeStr=uint8
  Constant5 : Constant  Value=12  OutDataTypeStr=uint8
  Constant6 : Constant  OutDataTypeStr=uint8
  Constant9 : Constant  Value=1970  OutDataTypeStr=uint16
  Data Type Conversion : DataTypeConversion  OutDataTypeStr=uint8
  Data Type Conversion1 : DataTypeConversion  OutDataTypeStr=uint8
  Data Type Conversion2 : DataTypeConversion  OutDataTypeStr=uint8
  Logical Operator1 : Logic  Inputs=6  AllPortsSameDT=off  OutDataTypeStr=boolean
  Switch : Switch  Criteria=u2 ~= 0
  Switch1 : Switch  Criteria=u2 ~= 0
  u8_Seconds : Outport  OutDataTypeStr=uint8
  u8_Minutes : Outport  Port=2  OutDataTypeStr=uint8
  u8_Hours : Outport  Port=3  OutDataTypeStr=uint8
  u8_Day : Outport  Port=4  OutDataTypeStr=uint8
  u8_Month : Outport  Port=5  OutDataTypeStr=uint8
  u16_Year : Outport  Port=6  OutDataTypeStr=uint16
  bo_ENO : Outport  Port=7  OutDataTypeStr=boolean
  wires:
  u16_YearIn/1 -> CheckIfYearIsValid/1(u16_YearIn), CheckIfDayIsValid/3(u16_YearIn), [u16_YearIn]
  Constant/1 -> Bus Creator/6, CheckIfYearIsValid/3(u16_MaxYear)  "u16_Year"
  u8_HoursIn/1 -> Bus Creator2/3, CheckIfHoursAreValid/1(u8_HoursIn)  "u8_Hours"
  u8_MinutesIn/1 -> Bus Creator2/2, CheckIfMinutesAreValid/1(u8_MinutesIn)  "u8_Minutes"
  u8_SecondsIn/1 -> CheckIfSecondsAreValid/1(u8_SecondsIn), Bus Creator2/1  "u8_Seconds"
  u8_DayIn/1 -> Bus Creator2/4, CheckIfDayIsValid/1(u8_DayIn)  "u8_Day"
  Constant5/1 -> CheckIfMonthIsValid/2(u8_MaxMonth), [u8_MaxMonth]
  CheckIfMinutesAreValid/1(bo_AreMinutesValid) -> Logical Operator1/2
  CheckIfHoursAreValid/1(bo_AreHoursValid) -> Logical Operator1/3
  Constant9/1 -> [u16_MinYear], CheckIfYearIsValid/2(u16_MinYear)
  Constant11/1 -> Bus Creator/7  "bo_ENO"
  [u8_MaxMinutes] -> Bus Creator/2  "u8_Minutes"
  [u8_MaxHours] -> Bus Creator/3  "u8_Hours"
  Constant3/1 -> CheckIfHoursAreValid/2(u8_MaxHours), [u8_MaxHours]
  Constant10/1 -> Bus Creator/4  "u8_Day"
  [u8_MaxMonth] -> Bus Creator/5  "u8_Month"
  [u8_MinMonth] -> Bus Creator1/5  "u8_Month"
  Logical Operator1/1 -> Switch1/2
  Bus Creator1/1 -> Switch1/3  "st_MinDate"
  [u8_MonthIn] -> Bus Creator2/5  "u8_Month"
  [u16_YearIn] -> Bus Creator2/6  "u16_Year"
  Constant13/1 -> Bus Creator1/7  "bo_ENO"
  Bus Selector/4 -> u8_Day/1  "<u8_Day>"
  Bus Selector/3 -> u8_Hours/1  "<u8_Hours>"
  Bus Selector/2 -> u8_Minutes/1  "<u8_Minutes>"
  Bus Selector/1 -> u8_Seconds/1  "<u8_Seconds>"
  Bus Selector/6 -> u16_Year/1  "<u16_Year>"
  Bus Selector/7 -> bo_ENO/1  "<bo_ENO>"
  Bus Creator2/1 -> Switch1/1  "st_OriginalDate"
  Switch1/1 -> Switch/1
  Bus Creator/1 -> Switch/3  "st_MaxDate"
  Switch/1 -> Bus Selector/1  "st_ValidDate"
  Constant14/1 -> Bus Creator2/7  "bo_ENO"
  Data Type Conversion/1 -> Bus Creator1/1  "u8_Seconds"
  [u8_MinDay] -> Bus Creator1/4  "u8_Day"
  Constant15/1 -> Data Type Conversion2/1, Data Type Conversion1/1, Data Type Conversion/1
  [u8_MaxSeconds] -> Bus Creator/1  "u8_Seconds"
  Bus Selector/5 -> u8_Month/1  "<u8_Month>"
  u8_MonthIn/1 -> CheckIfDayIsValid/2(u8_MonthIn), [u8_MonthIn], CheckIfMonthIsValid/1(u8_Month)
  CheckIfDayIsValid/1(bo_IsDayValid) -> Logical Operator1/4
  Constant1/1 -> [u8_MaxSeconds], CheckIfSecondsAreValid/2(u8_MaxSeconds)
  CheckIfSecondsAreValid/1(bo_AreSecondsValid) -> Logical Operator1/1
  Constant2/1 -> [u8_MaxMinutes], CheckIfMinutesAreValid/2(u8_MaxMinutes)
  CheckIfMonthIsValid/1(bo_IsMonthValid) -> CheckIfDayIsValid/5(bo_IsMonthValid), Logical Operator1/5
  CheckIfYearIsValid/1(bo_IsGreaterOrEqualMin) -> Logical Operator1/6
  CheckIfYearIsValid/2(bo_IsLessOrEqualMax) -> Switch/2
  Constant4/1 -> [u8_MinMonth], CheckIfMonthIsValid/3(u8_MinMonth)
  Constant6/1 -> [u8_MinDay], CheckIfDayIsValid/4(u8_MinDay)
  [u16_MinYear] -> Bus Creator1/6  "u16_Year"
  Data Type Conversion1/1 -> Bus Creator1/2  "u8_Minutes"
  Data Type Conversion2/1 -> Bus Creator1/3  "u8_Hours"

== system APP_MyApplication/Model/APP_MyApplication_/DateTime/DateTimeAssemble/ConvertToDateTime ==
  u8_Seconds : Inport  OutDataTypeStr=uint8
  u8_Minutes : Inport  Port=2  OutDataTypeStr=uint8
  u8_Hours : Inport  Port=3  OutDataTypeStr=uint8
  u16_NrOfDays : Inport  Port=4  OutDataTypeStr=uint16
  Add : Sum  Inputs=++++  OutDataTypeStr=uint32
  ConvertDaysToSeconds : Subsystem
  ConvertHoursToSeconds : Subsystem
  ConvertMinutesToSeconds : Subsystem
  u32_DateTime : Outport  OutDataTypeStr=uint32
  wires:
  u8_Seconds/1 -> Add/1
  Add/1 -> u32_DateTime/1
  ConvertMinutesToSeconds/1(u16_SecFromMins) -> Add/2
  ConvertHoursToSeconds/1(u32_SecFromHrs) -> Add/3
  ConvertDaysToSeconds/1(u32_SecFromDays) -> Add/4
  u8_Minutes/1 -> ConvertMinutesToSeconds/1(u8_Minutes)
  u8_Hours/1 -> ConvertHoursToSeconds/1(u8_Hours)
  u16_NrOfDays/1 -> ConvertDaysToSeconds/1(u16_NrOfDays)

== system APP_MyApplication/Model/APP_MyApplication_/DateTime/DateTimeAssemble/ConvertToNrOfDays ==
  note: Convert to number of days
  u8_Day : Inport  OutDataTypeStr=uint8
  u8_Month : Inport  Port=2  OutDataTypeStr=uint8
  u16_Year : Inport  Port=3  OutDataTypeStr=uint16
  AddDays : Subsystem
  AddDaysForCompleteMonths : Subsystem  TreatAsAtomicUnit=on
  AddDaysForCompleteYears : Subsystem
  CheckIfDateInLeapYearBeforeMarch : Subsystem
  Subtract2 : Sum  Inputs=+++-  OutDataTypeStr=uint16
  u16_NrOfDays : Outport  OutDataTypeStr=uint16
  wires:
  u16_Year/1 -> CheckIfDateInLeapYearBeforeMarch/2(u16_Year), AddDaysForCompleteYears/1(u16_Year)
  Subtract2/1 -> u16_NrOfDays/1
  u8_Month/1 -> CheckIfDateInLeapYearBeforeMarch/1(u8_Month), AddDaysForCompleteMonths/1(u8_Month)
  u8_Day/1 -> AddDays/1(u8_Day)
  AddDaysForCompleteMonths/1(u16_DaysForMonths) -> Subtract2/2
  AddDays/1(u8_CompleteDays) -> Subtract2/1
  AddDaysForCompleteYears/1(u16_DaysForYears) -> Subtract2/3
  CheckIfDateInLeapYearBeforeMarch/1(bo_MinusOne) -> Subtract2/4
